simulink model "lab1ex3"  (R2024a)
settings: Solver=VariableStepAuto  StartTime=0.0  StopTime=50  MaxStep=0.001  RelTol=1e-3
libraries: dspfdesign x1

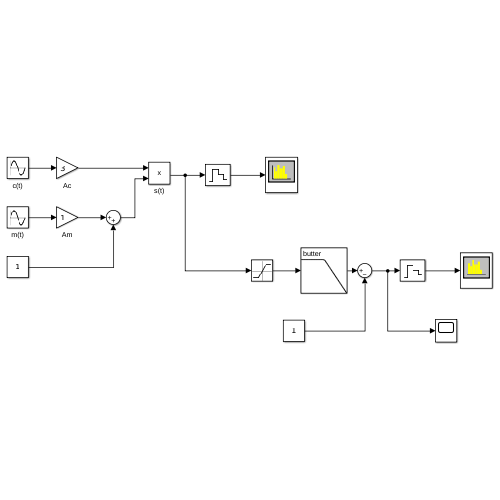
[thumbnail: Simulink's stored preview of the top-level diagram]
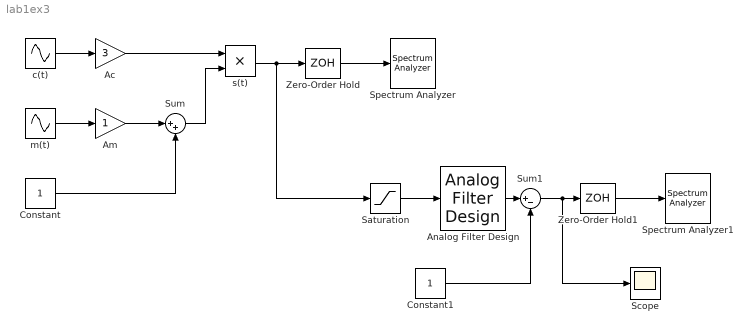
== system lab1ex3 ==
  Ac : Gain  Gain=3
  Am : Gain
  Analog Filter Design : dspfdesign/Analog Filter Design  method=Butterworth  filttype=Lowpass  N=8  Wlo=2*pi*2  Whi=80  Rp=2  Rs=40
  Constant : Constant
  Constant1 : Constant
  Saturation : Saturate  UpperLimit=10  LowerLimit=0
  Scope : Scope
  Spectrum Analyzer : SpectrumAnalyzer  WindowPosition=[436.000000,-240.000000,800.000000,500.000000,]  Visible=on  ScopeFrameLocation=window  ViewType=Spectrum and spectrogram  SpectrumUnits=Watts  YLimits=[-0.24586519,2.21288984]  ColorLimits=[-0.24586519,2.21288984]
  Spectrum Analyzer1 : SpectrumAnalyzer  WindowPosition=[284.000000,8.000000,800.000000,500.000000,]  ScopeFrameLocation=window  PlotAsTwoSidedSpectrum=off  SpectrumUnits=Watts  YLimits=[-0.01363696,0.12273522]  ColorLimits=[-0.10915491,0.9824002]  SelectedToolstripTab=spectrumAnalyzerToolstrip.spectrumTab
  Sum : Sum  Inputs=|++
  Sum1 : Sum  Inputs=|+-
  Zero-Order Hold : ZeroOrderHold  SampleTime=1/50
  Zero-Order Hold1 : ZeroOrderHold  SampleTime=1/50
  c(t) : Sin  Frequency=2*pi*10  Phase=pi/2  SampleTime=0
  m(t) : Sin  Frequency=2*pi*2  Phase=pi/2  SampleTime=0
  s(t) : Product
  wires:
  Am/1 -> Sum/1
  Constant/1 -> Sum/2
  Sum/1 -> s(t)/2
  Ac/1 -> s(t)/1
  c(t)/1 -> Ac/1
  m(t)/1 -> Am/1
  s(t)/1 -> Saturation/1, Zero-Order Hold/1
  Zero-Order Hold/1 -> Spectrum Analyzer/1
  Saturation/1 -> Analog Filter Design/1
  Zero-Order Hold1/1 -> Spectrum Analyzer1/1
  Analog Filter Design/1 -> Sum1/1
  Sum1/1 -> Scope/1, Zero-Order Hold1/1
  Constant1/1 -> Sum1/2
